simulink model "Robot"  (R2022b)
settings: Solver=FixedStepDiscrete  StartTime=0.0  StopTime=30  FixedStep=0.001  RelTol=1e-3
InitFcn:
  | load("BusConfig.mat");
undefined symbols (not defined in the file or in its folder): DiscIntNeverNeededParam
libraries: slrealtimeethercatlib x119, simulink x20
(part 7 of 7)

== system Robot/Subsystem/Robot/STM32Device2 ==
  EtherCAT PDO Receive1 : slrealtimeethercatlib/EtherCAT PDO Receive  Priority=2  sig_name=Box 6 (PIC32 EtherCAT Slave01).INPUTS process data mapping.FORCE1  sig_offset=37712  sig_type=single  type_size=32  sig_dim=1  device_id=0  sample_time=0.001000
  EtherCAT PDO Receive2 : slrealtimeethercatlib/EtherCAT PDO Receive  Priority=2  sig_name=Box 6 (PIC32 EtherCAT Slave01).INPUTS process data mapping.FORCE2  sig_offset=37744  sig_type=single  type_size=32  sig_dim=1  device_id=0  sample_time=0.001000
  EtherCAT PDO Receive3 : slrealtimeethercatlib/EtherCAT PDO Receive  Priority=2  sig_name=Box 6 (PIC32 EtherCAT Slave01).INPUTS process data mapping.IMU1_X  sig_offset=37968  sig_type=single  type_size=32  sig_dim=1  device_id=0  sample_time=0.001000
  EtherCAT PDO Receive4 : slrealtimeethercatlib/EtherCAT PDO Receive  Priority=2  sig_name=Box 6 (PIC32 EtherCAT Slave01).INPUTS process data mapping.IMU1_Y  sig_offset=38000  sig_type=single  type_size=32  sig_dim=1  device_id=0  sample_time=0.001000
  EtherCAT PDO Receive5 : slrealtimeethercatlib/EtherCAT PDO Receive  Priority=2  sig_name=Box 6 (PIC32 EtherCAT Slave01).INPUTS process data mapping.IMU1_Z  sig_offset=38032  sig_type=single  type_size=32  sig_dim=1  device_id=0  sample_time=0.001000
  EtherCAT PDO Receive6 : slrealtimeethercatlib/EtherCAT PDO Receive  Priority=2  sig_name=Box 6 (PIC32 EtherCAT Slave01).INPUTS process data mapping.IMU2_X  sig_offset=38064  sig_type=single  type_size=32  sig_dim=1  device_id=0  sample_time=0.001000
  AD_Ch1 : Outport
  AD_Ch2 : Outport  Port=2
  Quaternions_q0 : Outport  Port=3
  Quaternions_q1 : Outport  Port=4
  Quaternions_q2 : Outport  Port=5
  Quaternions_q3 : Outport  Port=6
  wires:
  EtherCAT PDO Receive1/1 -> AD_Ch1/1
  EtherCAT PDO Receive4/1 -> Quaternions_q1/1
  EtherCAT PDO Receive5/1 -> Quaternions_q2/1
  EtherCAT PDO Receive3/1 -> Quaternions_q0/1
  EtherCAT PDO Receive6/1 -> Quaternions_q3/1
  EtherCAT PDO Receive2/1 -> AD_Ch2/1

== system Robot/Subsystem/Robot/STM32Device3 ==
  EtherCAT PDO Receive1 : slrealtimeethercatlib/EtherCAT PDO Receive  Priority=2  sig_name=Box 7 (PIC32 EtherCAT Slave01).INPUTS process data mapping.FORCE1  sig_offset=38352  sig_type=single  type_size=32  sig_dim=1  device_id=0  sample_time=0.001000
  EtherCAT PDO Receive2 : slrealtimeethercatlib/EtherCAT PDO Receive  Priority=2  sig_name=Box 7 (PIC32 EtherCAT Slave01).INPUTS process data mapping.FORCE2  sig_offset=38384  sig_type=single  type_size=32  sig_dim=1  device_id=0  sample_time=0.001000
  EtherCAT PDO Receive3 : slrealtimeethercatlib/EtherCAT PDO Receive  Priority=2  sig_name=Box 7 (PIC32 EtherCAT Slave01).INPUTS process data mapping.IMU1_X  sig_offset=38608  sig_type=single  type_size=32  sig_dim=1  device_id=0  sample_time=0.001000
  EtherCAT PDO Receive4 : slrealtimeethercatlib/EtherCAT PDO Receive  Priority=2  sig_name=Box 7 (PIC32 EtherCAT Slave01).INPUTS process data mapping.IMU1_Y  sig_offset=38640  sig_type=single  type_size=32  sig_dim=1  device_id=0  sample_time=0.001000
  EtherCAT PDO Receive5 : slrealtimeethercatlib/EtherCAT PDO Receive  Priority=2  sig_name=Box 7 (PIC32 EtherCAT Slave01).INPUTS process data mapping.IMU1_Z  sig_offset=38672  sig_type=single  type_size=32  sig_dim=1  device_id=0  sample_time=0.001000
  EtherCAT PDO Receive6 : slrealtimeethercatlib/EtherCAT PDO Receive  Priority=2  sig_name=Box 7 (PIC32 EtherCAT Slave01).INPUTS process data mapping.IMU2_X  sig_offset=38704  sig_type=single  type_size=32  sig_dim=1  device_id=0  sample_time=0.001000
  AD_Ch1 : Outport
  AD_Ch2 : Outport  Port=2
  Quaternions_q0 : Outport  Port=3
  Quaternions_q1 : Outport  Port=4
  Quaternions_q2 : Outport  Port=5
  Quaternions_q3 : Outport  Port=6
  wires:
  EtherCAT PDO Receive1/1 -> AD_Ch1/1
  EtherCAT PDO Receive4/1 -> Quaternions_q1/1
  EtherCAT PDO Receive5/1 -> Quaternions_q2/1
  EtherCAT PDO Receive3/1 -> Quaternions_q0/1
  EtherCAT PDO Receive6/1 -> Quaternions_q3/1
  EtherCAT PDO Receive2/1 -> AD_Ch2/1

== system Robot/Motor1 Torque Control Init Frame/State_10_Enable/Subsystem/Switch Case Action Subsystem ==
  In1 : Inport
  Action Port : ActionPort  ActionPortLabel=case [ 10 ]:
  Out1 : Outport
  wires:
  In1/1 -> Out1/1

== system Robot/Motor1 Torque Control Init Frame/State_10_Enable/Subsystem/Switch Case Action Subsystem1 ==
  In1 : Inport
  Action Port : ActionPort  ActionPortLabel=default:
  Default : Outport
  wires:
  In1/1 -> Default/1

== system Robot/Motor1 Torque Control Init Frame/State_11_Enable/Subsystem/Switch Case Action Subsystem ==
  In1 : Inport
  Action Port : ActionPort  ActionPortLabel=case [ 11 ]:
  Out1 : Outport
  wires:
  In1/1 -> Out1/1

== system Robot/Motor1 Torque Control Init Frame/State_11_Enable/Subsystem/Switch Case Action Subsystem1 ==
  In1 : Inport
  Action Port : ActionPort  ActionPortLabel=default:
  Default : Outport
  wires:
  In1/1 -> Default/1

== system Robot/Motor1 Torque Control Init Frame/State_12_Enable/Subsystem/Switch Case Action Subsystem ==
  In1 : Inport
  Action Port : ActionPort  ActionPortLabel=case [ 12 ]:
  Out1 : Outport
  wires:
  In1/1 -> Out1/1

== system Robot/Motor1 Torque Control Init Frame/State_12_Enable/Subsystem/Switch Case Action Subsystem1 ==
  In1 : Inport
  Action Port : ActionPort  ActionPortLabel=default:
  Default : Outport
  wires:
  In1/1 -> Default/1

== system Robot/Motor1 Torque Control Init Frame/State_13_Enable/Subsystem/Switch Case Action Subsystem ==
  In1 : Inport
  Action Port : ActionPort  ActionPortLabel=case [ 13 ]:
  Out1 : Outport
  wires:
  In1/1 -> Out1/1

== system Robot/Motor1 Torque Control Init Frame/State_13_Enable/Subsystem/Switch Case Action Subsystem1 ==
  In1 : Inport
  Action Port : ActionPort  ActionPortLabel=default:
  Default : Outport
  wires:
  In1/1 -> Default/1

== system Robot/Motor1 Torque Control Init Frame/State_1_Enable/Subsystem/Switch Case Action Subsystem ==
  In1 : Inport
  Action Port : ActionPort  ActionPortLabel=case [ 1 ]:
  Out1 : Outport
  wires:
  In1/1 -> Out1/1

== system Robot/Motor1 Torque Control Init Frame/State_1_Enable/Subsystem/Switch Case Action Subsystem1 ==
  In1 : Inport
  Action Port : ActionPort  ActionPortLabel=default:
  Default : Outport
  wires:
  In1/1 -> Default/1

== system Robot/Motor1 Torque Control Init Frame/State_2_Enable/Subsystem/Switch Case Action Subsystem ==
  In1 : Inport
  Action Port : ActionPort  ActionPortLabel=case [ 2 ]:
  Out1 : Outport
  wires:
  In1/1 -> Out1/1

== system Robot/Motor1 Torque Control Init Frame/State_2_Enable/Subsystem/Switch Case Action Subsystem1 ==
  In1 : Inport
  Action Port : ActionPort  ActionPortLabel=default:
  Default : Outport
  wires:
  In1/1 -> Default/1

== system Robot/Motor1 Torque Control Init Frame/State_3_Enable/Subsystem/Switch Case Action Subsystem ==
  In1 : Inport
  Action Port : ActionPort  ActionPortLabel=case [ 3 ]:
  Out1 : Outport
  wires:
  In1/1 -> Out1/1

== system Robot/Motor1 Torque Control Init Frame/State_3_Enable/Subsystem/Switch Case Action Subsystem1 ==
  In1 : Inport
  Action Port : ActionPort  ActionPortLabel=default:
  Default : Outport
  wires:
  In1/1 -> Default/1

== system Robot/Motor1 Torque Control Init Frame/State_4_Enable/Subsystem/Switch Case Action Subsystem ==
  In1 : Inport
  Action Port : ActionPort  ActionPortLabel=case [ 4 ]:
  Out1 : Outport
  wires:
  In1/1 -> Out1/1

== system Robot/Motor1 Torque Control Init Frame/State_4_Enable/Subsystem/Switch Case Action Subsystem1 ==
  In1 : Inport
  Action Port : ActionPort  ActionPortLabel=default:
  Default : Outport
  wires:
  In1/1 -> Default/1

== system Robot/Motor1 Torque Control Init Frame/State_5_Enable/Subsystem/Switch Case Action Subsystem ==
  In1 : Inport
  Action Port : ActionPort  ActionPortLabel=case [ 5 ]:
  Out1 : Outport
  wires:
  In1/1 -> Out1/1

== system Robot/Motor1 Torque Control Init Frame/State_5_Enable/Subsystem/Switch Case Action Subsystem1 ==
  In1 : Inport
  Action Port : ActionPort  ActionPortLabel=default:
  Default : Outport
  wires:
  In1/1 -> Default/1

== system Robot/Motor1 Torque Control Init Frame/State_6_Enable/Subsystem/Switch Case Action Subsystem ==
  In1 : Inport
  Action Port : ActionPort  ActionPortLabel=case [ 6 ]:
  Out1 : Outport
  wires:
  In1/1 -> Out1/1

== system Robot/Motor1 Torque Control Init Frame/State_6_Enable/Subsystem/Switch Case Action Subsystem1 ==
  In1 : Inport
  Action Port : ActionPort  ActionPortLabel=default:
  Default : Outport
  wires:
  In1/1 -> Default/1

== system Robot/Motor1 Torque Control Init Frame/State_7_Enable/Subsystem/Switch Case Action Subsystem ==
  In1 : Inport
  Action Port : ActionPort  ActionPortLabel=case [ 7 ]:
  Out1 : Outport
  wires:
  In1/1 -> Out1/1

== system Robot/Motor1 Torque Control Init Frame/State_7_Enable/Subsystem/Switch Case Action Subsystem1 ==
  In1 : Inport
  Action Port : ActionPort  ActionPortLabel=default:
  Default : Outport
  wires:
  In1/1 -> Default/1

== system Robot/Motor1 Torque Control Init Frame/State_8_Enable/Subsystem/Switch Case Action Subsystem ==
  In1 : Inport
  Action Port : ActionPort  ActionPortLabel=case [ 8 ]:
  Out1 : Outport
  wires:
  In1/1 -> Out1/1

== system Robot/Motor1 Torque Control Init Frame/State_8_Enable/Subsystem/Switch Case Action Subsystem1 ==
  In1 : Inport
  Action Port : ActionPort  ActionPortLabel=default:
  Default : Outport
  wires:
  In1/1 -> Default/1

== system Robot/Motor1 Torque Control Init Frame/State_9_Enable/Subsystem/Switch Case Action Subsystem ==
  In1 : Inport
  Action Port : ActionPort  ActionPortLabel=case [ 9 ]:
  Out1 : Outport
  wires:
  In1/1 -> Out1/1

== system Robot/Motor1 Torque Control Init Frame/State_9_Enable/Subsystem/Switch Case Action Subsystem1 ==
  In1 : Inport
  Action Port : ActionPort  ActionPortLabel=default:
  Default : Outport
  wires:
  In1/1 -> Default/1

== system Robot/Motor2 Torque Control Init Frame/State_10_Enable/Subsystem/Switch Case Action Subsystem ==
  In1 : Inport
  Action Port : ActionPort  ActionPortLabel=case [ 10 ]:
  Out1 : Outport
  wires:
  In1/1 -> Out1/1

== system Robot/Motor2 Torque Control Init Frame/State_10_Enable/Subsystem/Switch Case Action Subsystem1 ==
  In1 : Inport
  Action Port : ActionPort  ActionPortLabel=default:
  Default : Outport
  wires:
  In1/1 -> Default/1

== system Robot/Motor2 Torque Control Init Frame/State_11_Enable/Subsystem/Switch Case Action Subsystem ==
  In1 : Inport
  Action Port : ActionPort  ActionPortLabel=case [ 11 ]:
  Out1 : Outport
  wires:
  In1/1 -> Out1/1

== system Robot/Motor2 Torque Control Init Frame/State_11_Enable/Subsystem/Switch Case Action Subsystem1 ==
  In1 : Inport
  Action Port : ActionPort  ActionPortLabel=default:
  Default : Outport
  wires:
  In1/1 -> Default/1

== system Robot/Motor2 Torque Control Init Frame/State_12_Enable/Subsystem/Switch Case Action Subsystem ==
  In1 : Inport
  Action Port : ActionPort  ActionPortLabel=case [ 12 ]:
  Out1 : Outport
  wires:
  In1/1 -> Out1/1

== system Robot/Motor2 Torque Control Init Frame/State_12_Enable/Subsystem/Switch Case Action Subsystem1 ==
  In1 : Inport
  Action Port : ActionPort  ActionPortLabel=default:
  Default : Outport
  wires:
  In1/1 -> Default/1

== system Robot/Motor2 Torque Control Init Frame/State_13_Enable/Subsystem/Switch Case Action Subsystem ==
  In1 : Inport
  Action Port : ActionPort  ActionPortLabel=case [ 13 ]:
  Out1 : Outport
  wires:
  In1/1 -> Out1/1

== system Robot/Motor2 Torque Control Init Frame/State_13_Enable/Subsystem/Switch Case Action Subsystem1 ==
  In1 : Inport
  Action Port : ActionPort  ActionPortLabel=default:
  Default : Outport
  wires:
  In1/1 -> Default/1

== system Robot/Motor2 Torque Control Init Frame/State_1_Enable/Subsystem/Switch Case Action Subsystem ==
  In1 : Inport
  Action Port : ActionPort  ActionPortLabel=case [ 1 ]:
  Out1 : Outport
  wires:
  In1/1 -> Out1/1

== system Robot/Motor2 Torque Control Init Frame/State_1_Enable/Subsystem/Switch Case Action Subsystem1 ==
  In1 : Inport
  Action Port : ActionPort  ActionPortLabel=default:
  Default : Outport
  wires:
  In1/1 -> Default/1

== system Robot/Motor2 Torque Control Init Frame/State_2_Enable/Subsystem/Switch Case Action Subsystem ==
  In1 : Inport
  Action Port : ActionPort  ActionPortLabel=case [ 2 ]:
  Out1 : Outport
  wires:
  In1/1 -> Out1/1

== system Robot/Motor2 Torque Control Init Frame/State_2_Enable/Subsystem/Switch Case Action Subsystem1 ==
  In1 : Inport
  Action Port : ActionPort  ActionPortLabel=default:
  Default : Outport
  wires:
  In1/1 -> Default/1

== system Robot/Motor2 Torque Control Init Frame/State_3_Enable/Subsystem/Switch Case Action Subsystem ==
  In1 : Inport
  Action Port : ActionPort  ActionPortLabel=case [ 3 ]:
  Out1 : Outport
  wires:
  In1/1 -> Out1/1

== system Robot/Motor2 Torque Control Init Frame/State_3_Enable/Subsystem/Switch Case Action Subsystem1 ==
  In1 : Inport
  Action Port : ActionPort  ActionPortLabel=default:
  Default : Outport
  wires:
  In1/1 -> Default/1

== system Robot/Motor2 Torque Control Init Frame/State_4_Enable/Subsystem/Switch Case Action Subsystem ==
  In1 : Inport
  Action Port : ActionPort  ActionPortLabel=case [ 4 ]:
  Out1 : Outport
  wires:
  In1/1 -> Out1/1

== system Robot/Motor2 Torque Control Init Frame/State_4_Enable/Subsystem/Switch Case Action Subsystem1 ==
  In1 : Inport
  Action Port : ActionPort  ActionPortLabel=default:
  Default : Outport
  wires:
  In1/1 -> Default/1

== system Robot/Motor2 Torque Control Init Frame/State_5_Enable/Subsystem/Switch Case Action Subsystem ==
  In1 : Inport
  Action Port : ActionPort  ActionPortLabel=case [ 5 ]:
  Out1 : Outport
  wires:
  In1/1 -> Out1/1

== system Robot/Motor2 Torque Control Init Frame/State_5_Enable/Subsystem/Switch Case Action Subsystem1 ==
  In1 : Inport
  Action Port : ActionPort  ActionPortLabel=default:
  Default : Outport
  wires:
  In1/1 -> Default/1

== system Robot/Motor2 Torque Control Init Frame/State_6_Enable/Subsystem/Switch Case Action Subsystem ==
  In1 : Inport
  Action Port : ActionPort  ActionPortLabel=case [ 6 ]:
  Out1 : Outport
  wires:
  In1/1 -> Out1/1

== system Robot/Motor2 Torque Control Init Frame/State_6_Enable/Subsystem/Switch Case Action Subsystem1 ==
  In1 : Inport
  Action Port : ActionPort  ActionPortLabel=default:
  Default : Outport
  wires:
  In1/1 -> Default/1

== system Robot/Motor2 Torque Control Init Frame/State_7_Enable/Subsystem/Switch Case Action Subsystem ==
  In1 : Inport
  Action Port : ActionPort  ActionPortLabel=case [ 7 ]:
  Out1 : Outport
  wires:
  In1/1 -> Out1/1

== system Robot/Motor2 Torque Control Init Frame/State_7_Enable/Subsystem/Switch Case Action Subsystem1 ==
  In1 : Inport
  Action Port : ActionPort  ActionPortLabel=default:
  Default : Outport
  wires:
  In1/1 -> Default/1

== system Robot/Motor2 Torque Control Init Frame/State_8_Enable/Subsystem/Switch Case Action Subsystem ==
  In1 : Inport
  Action Port : ActionPort  ActionPortLabel=case [ 8 ]:
  Out1 : Outport
  wires:
  In1/1 -> Out1/1

== system Robot/Motor2 Torque Control Init Frame/State_8_Enable/Subsystem/Switch Case Action Subsystem1 ==
  In1 : Inport
  Action Port : ActionPort  ActionPortLabel=default:
  Default : Outport
  wires:
  In1/1 -> Default/1

== system Robot/Motor2 Torque Control Init Frame/State_9_Enable/Subsystem/Switch Case Action Subsystem ==
  In1 : Inport
  Action Port : ActionPort  ActionPortLabel=case [ 9 ]:
  Out1 : Outport
  wires:
  In1/1 -> Out1/1

== system Robot/Motor2 Torque Control Init Frame/State_9_Enable/Subsystem/Switch Case Action Subsystem1 ==
  In1 : Inport
  Action Port : ActionPort  ActionPortLabel=default:
  Default : Outport
  wires:
  In1/1 -> Default/1

== system Robot/Motor3 Torque Control Init Frame/State_10_Enable/Subsystem/Switch Case Action Subsystem ==
  In1 : Inport
  Action Port : ActionPort  ActionPortLabel=case [ 10 ]:
  Out1 : Outport
  wires:
  In1/1 -> Out1/1

== system Robot/Motor3 Torque Control Init Frame/State_10_Enable/Subsystem/Switch Case Action Subsystem1 ==
  In1 : Inport
  Action Port : ActionPort  ActionPortLabel=default:
  Default : Outport
  wires:
  In1/1 -> Default/1

== system Robot/Motor3 Torque Control Init Frame/State_11_Enable/Subsystem/Switch Case Action Subsystem ==
  In1 : Inport
  Action Port : ActionPort  ActionPortLabel=case [ 11 ]:
  Out1 : Outport
  wires:
  In1/1 -> Out1/1

== system Robot/Motor3 Torque Control Init Frame/State_11_Enable/Subsystem/Switch Case Action Subsystem1 ==
  In1 : Inport
  Action Port : ActionPort  ActionPortLabel=default:
  Default : Outport
  wires:
  In1/1 -> Default/1

== system Robot/Motor3 Torque Control Init Frame/State_12_Enable/Subsystem/Switch Case Action Subsystem ==
  In1 : Inport
  Action Port : ActionPort  ActionPortLabel=case [ 12 ]:
  Out1 : Outport
  wires:
  In1/1 -> Out1/1

== system Robot/Motor3 Torque Control Init Frame/State_12_Enable/Subsystem/Switch Case Action Subsystem1 ==
  In1 : Inport
  Action Port : ActionPort  ActionPortLabel=default:
  Default : Outport
  wires:
  In1/1 -> Default/1

== system Robot/Motor3 Torque Control Init Frame/State_13_Enable/Subsystem/Switch Case Action Subsystem ==
  In1 : Inport
  Action Port : ActionPort  ActionPortLabel=case [ 13 ]:
  Out1 : Outport
  wires:
  In1/1 -> Out1/1

== system Robot/Motor3 Torque Control Init Frame/State_13_Enable/Subsystem/Switch Case Action Subsystem1 ==
  In1 : Inport
  Action Port : ActionPort  ActionPortLabel=default:
  Default : Outport
  wires:
  In1/1 -> Default/1

== system Robot/Motor3 Torque Control Init Frame/State_1_Enable/Subsystem/Switch Case Action Subsystem ==
  In1 : Inport
  Action Port : ActionPort  ActionPortLabel=case [ 1 ]:
  Out1 : Outport
  wires:
  In1/1 -> Out1/1

== system Robot/Motor3 Torque Control Init Frame/State_1_Enable/Subsystem/Switch Case Action Subsystem1 ==
  In1 : Inport
  Action Port : ActionPort  ActionPortLabel=default:
  Default : Outport
  wires:
  In1/1 -> Default/1

== system Robot/Motor3 Torque Control Init Frame/State_2_Enable/Subsystem/Switch Case Action Subsystem ==
  In1 : Inport
  Action Port : ActionPort  ActionPortLabel=case [ 2 ]:
  Out1 : Outport
  wires:
  In1/1 -> Out1/1

== system Robot/Motor3 Torque Control Init Frame/State_2_Enable/Subsystem/Switch Case Action Subsystem1 ==
  In1 : Inport
  Action Port : ActionPort  ActionPortLabel=default:
  Default : Outport
  wires:
  In1/1 -> Default/1

== system Robot/Motor3 Torque Control Init Frame/State_3_Enable/Subsystem/Switch Case Action Subsystem ==
  In1 : Inport
  Action Port : ActionPort  ActionPortLabel=case [ 3 ]:
  Out1 : Outport
  wires:
  In1/1 -> Out1/1

== system Robot/Motor3 Torque Control Init Frame/State_3_Enable/Subsystem/Switch Case Action Subsystem1 ==
  In1 : Inport
  Action Port : ActionPort  ActionPortLabel=default:
  Default : Outport
  wires:
  In1/1 -> Default/1

== system Robot/Motor3 Torque Control Init Frame/State_4_Enable/Subsystem/Switch Case Action Subsystem ==
  In1 : Inport
  Action Port : ActionPort
  Out1 : Outport
  wires:
  In1/1 -> Out1/1

== system Robot/Motor3 Torque Control Init Frame/State_4_Enable/Subsystem/Switch Case Action Subsystem1 ==
  In1 : Inport
  Action Port : ActionPort
  Default : Outport
  wires:
  In1/1 -> Default/1

== system Robot/Motor3 Torque Control Init Frame/State_5_Enable/Subsystem/Switch Case Action Subsystem ==
  In1 : Inport
  Action Port : ActionPort
  Out1 : Outport
  wires:
  In1/1 -> Out1/1

== system Robot/Motor3 Torque Control Init Frame/State_5_Enable/Subsystem/Switch Case Action Subsystem1 ==
  In1 : Inport
  Action Port : ActionPort
  Default : Outport
  wires:
  In1/1 -> Default/1

== system Robot/Motor3 Torque Control Init Frame/State_6_Enable/Subsystem/Switch Case Action Subsystem ==
  In1 : Inport
  Action Port : ActionPort
  Out1 : Outport
  wires:
  In1/1 -> Out1/1

== system Robot/Motor3 Torque Control Init Frame/State_6_Enable/Subsystem/Switch Case Action Subsystem1 ==
  In1 : Inport
  Action Port : ActionPort
  Default : Outport
  wires:
  In1/1 -> Default/1

== system Robot/Motor3 Torque Control Init Frame/State_7_Enable/Subsystem/Switch Case Action Subsystem ==
  In1 : Inport
  Action Port : ActionPort
  Out1 : Outport
  wires:
  In1/1 -> Out1/1

== system Robot/Motor3 Torque Control Init Frame/State_7_Enable/Subsystem/Switch Case Action Subsystem1 ==
  In1 : Inport
  Action Port : ActionPort
  Default : Outport
  wires:
  In1/1 -> Default/1

== system Robot/Motor3 Torque Control Init Frame/State_8_Enable/Subsystem/Switch Case Action Subsystem ==
  In1 : Inport
  Action Port : ActionPort
  Out1 : Outport
  wires:
  In1/1 -> Out1/1

== system Robot/Motor3 Torque Control Init Frame/State_8_Enable/Subsystem/Switch Case Action Subsystem1 ==
  In1 : Inport
  Action Port : ActionPort
  Default : Outport
  wires:
  In1/1 -> Default/1

== system Robot/Motor3 Torque Control Init Frame/State_9_Enable/Subsystem/Switch Case Action Subsystem ==
  In1 : Inport
  Action Port : ActionPort  ActionPortLabel=case [ 9 ]:
  Out1 : Outport
  wires:
  In1/1 -> Out1/1

== system Robot/Motor3 Torque Control Init Frame/State_9_Enable/Subsystem/Switch Case Action Subsystem1 ==
  In1 : Inport
  Action Port : ActionPort  ActionPortLabel=default:
  Default : Outport
  wires:
  In1/1 -> Default/1

== system Robot/Motor4 Torque Control Init Frame/State_10_Enable/Subsystem/Switch Case Action Subsystem ==
  In1 : Inport
  Action Port : ActionPort  ActionPortLabel=case [ 10 ]:
  Out1 : Outport
  wires:
  In1/1 -> Out1/1

== system Robot/Motor4 Torque Control Init Frame/State_10_Enable/Subsystem/Switch Case Action Subsystem1 ==
  In1 : Inport
  Action Port : ActionPort  ActionPortLabel=default:
  Default : Outport
  wires:
  In1/1 -> Default/1

== system Robot/Motor4 Torque Control Init Frame/State_11_Enable/Subsystem/Switch Case Action Subsystem ==
  In1 : Inport
  Action Port : ActionPort  ActionPortLabel=case [ 11 ]:
  Out1 : Outport
  wires:
  In1/1 -> Out1/1

== system Robot/Motor4 Torque Control Init Frame/State_11_Enable/Subsystem/Switch Case Action Subsystem1 ==
  In1 : Inport
  Action Port : ActionPort  ActionPortLabel=default:
  Default : Outport
  wires:
  In1/1 -> Default/1

== system Robot/Motor4 Torque Control Init Frame/State_12_Enable/Subsystem/Switch Case Action Subsystem ==
  In1 : Inport
  Action Port : ActionPort  ActionPortLabel=case [ 12 ]:
  Out1 : Outport
  wires:
  In1/1 -> Out1/1

== system Robot/Motor4 Torque Control Init Frame/State_12_Enable/Subsystem/Switch Case Action Subsystem1 ==
  In1 : Inport
  Action Port : ActionPort  ActionPortLabel=default:
  Default : Outport
  wires:
  In1/1 -> Default/1

== system Robot/Motor4 Torque Control Init Frame/State_13_Enable/Subsystem/Switch Case Action Subsystem ==
  In1 : Inport
  Action Port : ActionPort  ActionPortLabel=case [ 13 ]:
  Out1 : Outport
  wires:
  In1/1 -> Out1/1

== system Robot/Motor4 Torque Control Init Frame/State_13_Enable/Subsystem/Switch Case Action Subsystem1 ==
  In1 : Inport
  Action Port : ActionPort  ActionPortLabel=default:
  Default : Outport
  wires:
  In1/1 -> Default/1

== system Robot/Motor4 Torque Control Init Frame/State_1_Enable/Subsystem/Switch Case Action Subsystem ==
  In1 : Inport
  Action Port : ActionPort  ActionPortLabel=case [ 1 ]:
  Out1 : Outport
  wires:
  In1/1 -> Out1/1

== system Robot/Motor4 Torque Control Init Frame/State_1_Enable/Subsystem/Switch Case Action Subsystem1 ==
  In1 : Inport
  Action Port : ActionPort  ActionPortLabel=default:
  Default : Outport
  wires:
  In1/1 -> Default/1

== system Robot/Motor4 Torque Control Init Frame/State_2_Enable/Subsystem/Switch Case Action Subsystem ==
  In1 : Inport
  Action Port : ActionPort  ActionPortLabel=case [ 2 ]:
  Out1 : Outport
  wires:
  In1/1 -> Out1/1

== system Robot/Motor4 Torque Control Init Frame/State_2_Enable/Subsystem/Switch Case Action Subsystem1 ==
  In1 : Inport
  Action Port : ActionPort  ActionPortLabel=default:
  Default : Outport
  wires:
  In1/1 -> Default/1

== system Robot/Motor4 Torque Control Init Frame/State_3_Enable/Subsystem/Switch Case Action Subsystem ==
  In1 : Inport
  Action Port : ActionPort  ActionPortLabel=case [ 3 ]:
  Out1 : Outport
  wires:
  In1/1 -> Out1/1

== system Robot/Motor4 Torque Control Init Frame/State_3_Enable/Subsystem/Switch Case Action Subsystem1 ==
  In1 : Inport
  Action Port : ActionPort  ActionPortLabel=default:
  Default : Outport
  wires:
  In1/1 -> Default/1

== system Robot/Motor4 Torque Control Init Frame/State_4_Enable/Subsystem/Switch Case Action Subsystem ==
  In1 : Inport
  Action Port : ActionPort
  Out1 : Outport
  wires:
  In1/1 -> Out1/1

== system Robot/Motor4 Torque Control Init Frame/State_4_Enable/Subsystem/Switch Case Action Subsystem1 ==
  In1 : Inport
  Action Port : ActionPort
  Default : Outport
  wires:
  In1/1 -> Default/1

== system Robot/Motor4 Torque Control Init Frame/State_5_Enable/Subsystem/Switch Case Action Subsystem ==
  In1 : Inport
  Action Port : ActionPort
  Out1 : Outport
  wires:
  In1/1 -> Out1/1

== system Robot/Motor4 Torque Control Init Frame/State_5_Enable/Subsystem/Switch Case Action Subsystem1 ==
  In1 : Inport
  Action Port : ActionPort
  Default : Outport
  wires:
  In1/1 -> Default/1

== system Robot/Motor4 Torque Control Init Frame/State_6_Enable/Subsystem/Switch Case Action Subsystem ==
  In1 : Inport
  Action Port : ActionPort
  Out1 : Outport
  wires:
  In1/1 -> Out1/1

== system Robot/Motor4 Torque Control Init Frame/State_6_Enable/Subsystem/Switch Case Action Subsystem1 ==
  In1 : Inport
  Action Port : ActionPort
  Default : Outport
  wires:
  In1/1 -> Default/1

== system Robot/Motor4 Torque Control Init Frame/State_7_Enable/Subsystem/Switch Case Action Subsystem ==
  In1 : Inport
  Action Port : ActionPort
  Out1 : Outport
  wires:
  In1/1 -> Out1/1

== system Robot/Motor4 Torque Control Init Frame/State_7_Enable/Subsystem/Switch Case Action Subsystem1 ==
  In1 : Inport
  Action Port : ActionPort
  Default : Outport
  wires:
  In1/1 -> Default/1

== system Robot/Motor4 Torque Control Init Frame/State_8_Enable/Subsystem/Switch Case Action Subsystem ==
  In1 : Inport
  Action Port : ActionPort
  Out1 : Outport
  wires:
  In1/1 -> Out1/1

== system Robot/Motor4 Torque Control Init Frame/State_8_Enable/Subsystem/Switch Case Action Subsystem1 ==
  In1 : Inport
  Action Port : ActionPort
  Default : Outport
  wires:
  In1/1 -> Default/1

== system Robot/Motor4 Torque Control Init Frame/State_9_Enable/Subsystem/Switch Case Action Subsystem ==
  In1 : Inport
  Action Port : ActionPort  ActionPortLabel=case [ 9 ]:
  Out1 : Outport
  wires:
  In1/1 -> Out1/1

== system Robot/Motor4 Torque Control Init Frame/State_9_Enable/Subsystem/Switch Case Action Subsystem1 ==
  In1 : Inport
  Action Port : ActionPort  ActionPortLabel=default:
  Default : Outport
  wires:
  In1/1 -> Default/1

== stateflow chart Robot/Motor2 Torque Control Init Frame/Chart ==
  state Init_step0
    State=0;
    TaskFinished=0;
  state Init_step07
    State=7;
  state Init_step08
    State=8;
  state Init_step01
    State=1;
  state Init_step06
    State=6;
  state Init_step09
    State=9;
  state Init_step14
    State=14;
    TaskFinished=FinishIndex;
  state Init_step02
    State=2;
  state Init_step05
    State=5;
  state Init_step10
    State=10;
  state Init_step13
    State=13;
  state Init_step03
    State=3;
  state Init_step04
    State=4;
  state Init_step11
    State=11;
  state Init_step12
    State=12;
  (default) -> Init_step0
  Init_step07 -> Init_step08 : [TaskFinishedState==7]
  Init_step0 -> Init_step01
  Init_step06 -> Init_step07 : [TaskFinishedState==6]
  Init_step08 -> Init_step09 : [TaskFinishedState==8]
  Init_step01 -> Init_step02 : [TaskFinishedState==1]
  Init_step05 -> Init_step06 : [TaskFinishedState==5]
  Init_step09 -> ? : [TaskFinishedState==9]
  Init_step13 -> Init_step14 : [TaskFinishedState==13]
  Init_step03 -> Init_step10 : [TaskFinishedState==3]
  Init_step02 -> Init_step03 : [TaskFinishedState==2]
  Init_step04 -> Init_step05 : [TaskFinishedState==4]
  Init_step10 -> Init_step11 : [TaskFinishedState==10]
  Init_step12 -> Init_step13 : [TaskFinishedState==12]
  Init_step11 -> Init_step12 : [TaskFinishedState==11]
  data: FinishIndex input; State output; TaskFinishedState input; TaskFinished output

== stateflow chart Robot/Chart ==
  state Start
    State = 0;
  state InitMotor1
    State = 1;
  state InitMotor2
    State = 2;
  state InitMotor3
    State =3;
  state InitMotor4
    State=4;
  state Run
    State = 5;
  (default) -> Start
  Start -> InitMotor1 : [MasterState==8]
  InitMotor3 -> InitMotor4 : [TaskFinishedState==3]
  InitMotor4 -> Run : [TaskFinishedState==4]
  InitMotor1 -> InitMotor2 : [TaskFinishedState==1]
  InitMotor2 -> InitMotor3 : [TaskFinishedState==2]
  data: TaskFinishedState input; State output; MasterState input

== stateflow chart Robot/Motor3 Torque Control Init Frame/Chart ==
  state Init_step0
    State=0;
    TaskFinished=0;
  state Init_step07
    State=7;
  state Init_step08
    State=8;
  state Init_step01
    State=1;
  state Init_step06
    State=6;
  state Init_step09
    State=9;
  state Init_step14
    State=14;
    TaskFinished=FinishIndex;
  state Init_step02
    State=2;
  state Init_step05
    State=5;
  state Init_step10
    State=10;
  state Init_step13
    State=13;
  state Init_step03
    State=3;
  state Init_step04
    State=4;
  state Init_step11
    State=11;
  state Init_step12
    State=12;
  (default) -> Init_step0
  Init_step07 -> Init_step08 : [TaskFinishedState==7]
  Init_step0 -> Init_step01
  Init_step06 -> Init_step07 : [TaskFinishedState==6]
  Init_step08 -> Init_step09 : [TaskFinishedState==8]
  Init_step01 -> Init_step02 : [TaskFinishedState==1]
  Init_step05 -> Init_step06 : [TaskFinishedState==5]
  Init_step09 -> ? : [TaskFinishedState==9]
  Init_step13 -> Init_step14 : [TaskFinishedState==13]
  Init_step03 -> Init_step10 : [TaskFinishedState==3]
  Init_step02 -> Init_step03 : [TaskFinishedState==2]
  Init_step04 -> Init_step05 : [TaskFinishedState==4]
  Init_step10 -> Init_step11 : [TaskFinishedState==10]
  Init_step12 -> Init_step13 : [TaskFinishedState==12]
  Init_step11 -> Init_step12 : [TaskFinishedState==11]
  data: FinishIndex input; State output; TaskFinishedState input; TaskFinished output

== stateflow chart Robot/Motor4 Torque Control Init Frame/Chart ==
  state Init_step0
    State=0;
    TaskFinished=0;
  state Init_step07
    State=7;
  state Init_step08
    State=8;
  state Init_step01
    State=1;
  state Init_step06
    State=6;
  state Init_step09
    State=9;
  state Init_step14
    State=14;
    TaskFinished=FinishIndex;
  state Init_step02
    State=2;
  state Init_step05
    State=5;
  state Init_step10
    State=10;
  state Init_step13
    State=13;
  state Init_step03
    State=3;
  state Init_step04
    State=4;
  state Init_step11
    State=11;
  state Init_step12
    State=12;
  (default) -> Init_step0
  Init_step07 -> Init_step08 : [TaskFinishedState==7]
  Init_step0 -> Init_step01
  Init_step06 -> Init_step07 : [TaskFinishedState==6]
  Init_step08 -> Init_step09 : [TaskFinishedState==8]
  Init_step01 -> Init_step02 : [TaskFinishedState==1]
  Init_step05 -> Init_step06 : [TaskFinishedState==5]
  Init_step09 -> ? : [TaskFinishedState==9]
  Init_step13 -> Init_step14 : [TaskFinishedState==13]
  Init_step03 -> Init_step10 : [TaskFinishedState==3]
  Init_step02 -> Init_step03 : [TaskFinishedState==2]
  Init_step04 -> Init_step05 : [TaskFinishedState==4]
  Init_step10 -> Init_step11 : [TaskFinishedState==10]
  Init_step12 -> Init_step13 : [TaskFinishedState==12]
  Init_step11 -> Init_step12 : [TaskFinishedState==11]
  data: FinishIndex input; State output; TaskFinishedState input; TaskFinished output

== stateflow chart Robot/Motor1 Torque Control Init Frame/Chart ==
  state Init_step0
    State=0;
    TaskFinished=0;
  state Init_step07
    State=7;
  state Init_step08
    State=8;
  state Init_step01
    State=1;
  state Init_step06
    State=6;
  state Init_step09
    State=9;
  state Init_step14
    State=14;
    TaskFinished=FinishIndex;
  state Init_step02
    State=2;
  state Init_step05
    State=5;
  state Init_step10
    State=10;
  state Init_step13
    State=13;
  state Init_step03
    State=3;
  state Init_step04
    State=4;
  state Init_step11
    State=11;
  state Init_step12
    State=12;
  (default) -> Init_step0
  Init_step07 -> Init_step08 : [TaskFinishedState==7]
  Init_step0 -> Init_step01
  Init_step06 -> Init_step07 : [TaskFinishedState==6]
  Init_step08 -> Init_step09 : [TaskFinishedState==8]
  Init_step09 -> ? : [TaskFinishedState==9]
  Init_step01 -> Init_step02 : [TaskFinishedState==1]
  Init_step05 -> Init_step06 : [TaskFinishedState==5]
  Init_step13 -> Init_step14 : [TaskFinishedState==13]
  Init_step03 -> Init_step10 : [TaskFinishedState==3]
  Init_step02 -> Init_step03 : [TaskFinishedState==2]
  Init_step04 -> Init_step05 : [TaskFinishedState==4]
  Init_step10 -> Init_step11 : [TaskFinishedState==10]
  Init_step12 -> Init_step13 : [TaskFinishedState==12]
  Init_step11 -> Init_step12 : [TaskFinishedState==11]
  data: FinishIndex input; State output; TaskFinishedState input; TaskFinished output
